simulink model "satellite2"  (Simulink 7.5)
settings: Solver=ode45  StartTime=0.0  StopTime=10.0  RelTol=1e-3
libraries: simulink_extras x3, dspswit3 x3, commsynccomp2 x2, dspsrcs4 x1, commnoisgen2 x1
settings Model: Creator=sisa  LastModifiedBy=SISA

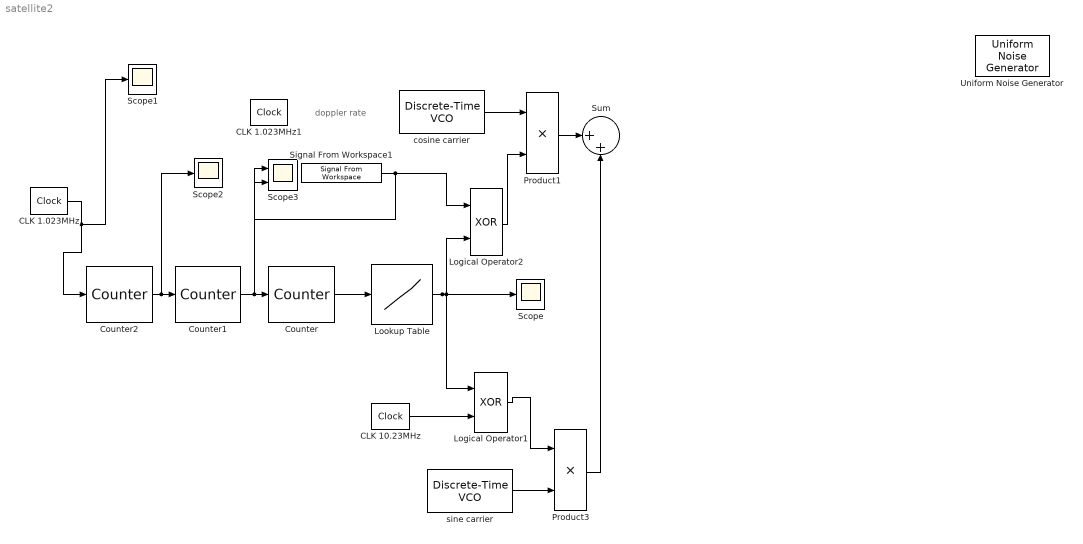
== system satellite2 ==
  note: doppler rate
  CLK 1.023MHz : simulink_extras/Flip Flops/Clock  SystemSampleTime=-1  MaskParam1=9.7751e-7
  CLK 1.023MHz1 : simulink_extras/Flip Flops/Clock  SystemSampleTime=-1  MaskParam1=9.7751e-7
  CLK 10.23MHz : simulink_extras/Flip Flops/Clock  SystemSampleTime=-1  MaskParam1=0.00000009775
  Counter : dspswit3/Counter  Direction=Up  CountEvent=Rising edge  CounterSize=User defined  MaxCount=1500  InitialCount=0  Output=Count  HitValue=32  ResetInput=off  SamplesPerFrame=1  Ts=1  CntDtype=double  HitDtype=Logical
  Counter1 : dspswit3/Counter  Direction=Up  CountEvent=Rising edge  CounterSize=User defined  MaxCount=20  InitialCount=0  Output=Count  HitValue=32  ResetInput=off  SamplesPerFrame=1  Ts=1  CntDtype=double  HitDtype=Logical
  Counter2 : dspswit3/Counter  Direction=Up  CountEvent=Falling edge  CounterSize=User defined  MaxCount=1022  InitialCount=0  Output=Count  HitValue=32  ResetInput=off  SamplesPerFrame=1  Ts=1  CntDtype=double  HitDtype=Logical
  Logical Operator1 : Logic  Operator=XOR  AllPortsSameDT=off  OutDataTypeMode=boolean  LogicDataType=fixdt(0, 8)  OutDataTypeStr=boolean
  Logical Operator2 : Logic  Operator=XOR  AllPortsSameDT=off  OutDataTypeMode=boolean  LogicDataType=fixdt(0, 8)  OutDataTypeStr=boolean
  Lookup Table : Lookup  InputValues=[-1,0,1]  Table=[-1,0,1]  LookUpMeth=Use Input Above  OutDataType=fixdt(1, 16)  OutScaling=2^0
  Product1 : Product  OutDataType=fixdt(1, 16)  OutScaling=2^0  RndMeth=Zero
  Product3 : Product  OutDataType=fixdt(1, 16)  OutScaling=2^0  RndMeth=Zero
  Scope : Scope
  Scope1 : Scope
  Scope2 : Scope
      settings: SaveName=ScopeData2
  Scope3 : Scope  NumInputPorts=2
      settings: YMin=-5~-5  YMax=5~5  SaveName=ScopeData3
  Signal From Workspace1 : dspsrcs4/Signal From Workspace  SystemSampleTime=-1  X=PN08  Ts=1  nsamps=1  OutputAfterFinalValue=Setting to zero  ignoreOrWarnInputAndFrameLengths=off
  Sum : Sum  Inputs=|++  OutDataType=fixdt(1, 16)  OutScaling=2^0
  Uniform Noise Generator : commnoisgen2/Uniform Noise Generator  SystemSampleTime=-1  low=0  up=1  seed=31  Ts=1  frameBased=off  sampPerFrame=1  orient=off  outDataType=double
  cosine carrier : commsynccomp2/Discrete-Time VCO  SystemSampleTime=-1  Ac=1  Fc=10e6  Kc=1  Ph=0  ts=0.01
  sine carrier : commsynccomp2/Discrete-Time VCO  SystemSampleTime=-1  Ac=1  Fc=10e6  Kc=1  Ph=0  ts=0.01
  wires:
  Lookup Table/1 -> Logical Operator2/2, Logical Operator1/1, Scope/1
  CLK 1.023MHz/1 -> Counter2/1, Scope1/1
  Counter2/1 -> Counter1/1, Scope2/1
  Counter1/1 -> Counter/1, Scope3/1
  Counter/1 -> Lookup Table/1
  sine carrier/1 -> Product3/2
  cosine carrier/1 -> Product1/1
  ? -> cosine carrier/1, sine carrier/1
  Product3/1 -> Sum/2
  Product1/1 -> Sum/1
  CLK 10.23MHz/1 -> Logical Operator1/2
  Signal From Workspace1/1 -> Logical Operator2/1, Scope3/2
  Logical Operator1/1 -> Product3/1
  Logical Operator2/1 -> Product1/2
